simulink model "svm"  (R2021b)
settings: Solver=VariableStepAuto  StartTime=0.0  StopTime=10.0  RelTol=1e-3
libraries: spsIGBTDiodeLib x6, slpidlib x2, spsAsynchronousMachineSIUnitsLib x1, spsDCVoltageSourceLib x1, mcbcontrolslib x1, simulink_extras x1, spsSeriesRLCBranchLib x1, spsTriangleGeneratorLib x1, spsVoltageMeasurementLib x1, spspowerguiLib x1
settings Model: Creator=borutzki  LastModifiedBy=borutzki

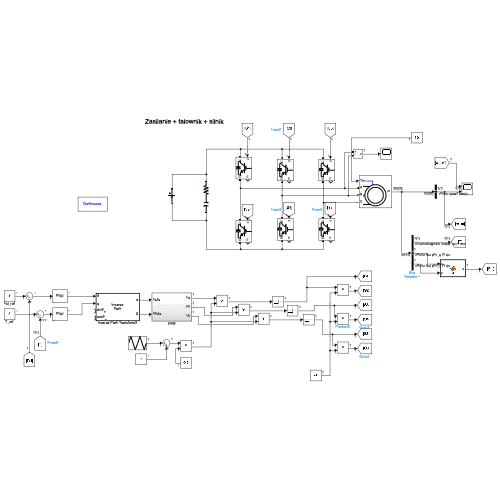
[thumbnail: Simulink's stored preview of the top-level diagram]
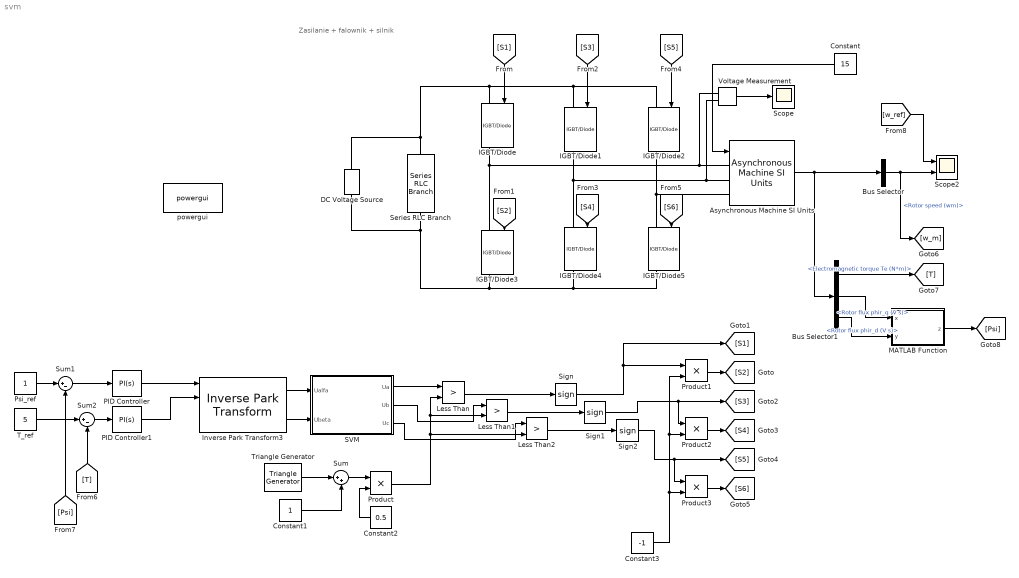
== system svm ==
  note: Zasilanie + falownik + silnik
  Asynchronous Machine SI Units : spsAsynchronousMachineSIUnitsLib/Asynchronous Machine SI Units  RotorType=Squirrel-cage  PresetModel=No  MechanicalLoad=Torque Tm  ShowDetailedParameters=on  ReferenceFrame=Rotor  Units=SI  MeasurementBus=off  NominalParameters=[1.845e+04 400 50]  VoltageRatio=1  Stator=[0.5968 0.0003495]  Rotor=[0.6258 0.005473]  Cage1=[0.4155 0.002066]  Cage2=[0.4168 0.0003495]  Lm=0.0354  Mechanical=[0.05 0.005879 2]  PolePairs=2  InitialConditions=[0 0 0 0 0 0 0 0]  SimulateSaturation=off  Saturation=[14.03593122, 27.81365428, 53.79336849, 72.68890987, 97.98006896, 148.6815601, 215.7428561, 302.9841135, 428.7778367 ; 230, 322, 414, 460, 506, 552, 598, 644, 690]  LoadFlowParameters=1492000  TsPowergui=0  TsBlock=-1  IterativeModel=Trapezoidal non iterative  IterativeDiscreteModel=Trapezoidal non iterative  Pmec=1.492e+006
  Bus Selector : BusSelector  OutputSignals=Mechanical.Rotor speed (wm)
  Bus Selector1 : BusSelector  OutputSignals=Mechanical.Electromagnetic torque Te (N*m),Rotor measurements.Rotor flux phir_q (V s),Rotor measurements.Rotor flux phir_d (V s)
  Constant : Constant  Value=15
  Constant1 : Constant
  Constant2 : Constant  Value=0.5
  Constant3 : Constant  Value=-1
  DC Voltage Source : spsDCVoltageSourceLib/DC Voltage Source  Amplitude=400  Measurements=None
  IGBT/Diode{,1..5} (6 alike) : spsIGBTDiodeLib/IGBT//Diode  Ron=1e-3  Rs=1e5  Cs=inf  Measurements=on
  Inverse Park Transform3 : mcbcontrolslib/Inverse Park Transform  AxisAlignment=D-axis
  Less Than : RelationalOperator  Operator=>  OutDataTypeStr=boolean  RndMeth=Simplest
  Less Than1 : RelationalOperator  Operator=>  OutDataTypeStr=boolean  RndMeth=Simplest
  Less Than2 : RelationalOperator  Operator=>  OutDataTypeStr=boolean  RndMeth=Simplest
  MATLAB Function : MATLAB Function  TreatAsAtomicUnit=on
  PID Controller : slpidlib/PID Controller  Controller=PI  Form=Parallel  TimeDomain=Continuous-time  UseExternalTs=off  SampleTime=-1  IntegratorMethod=Forward Euler  FilterMethod=Forward Euler  ControllerParametersSource=internal  P=1  I=1  D=0  UseFilter=on  N=100  TunerSelectOption=Transfer Function Based (PID Tuner App)  InitialConditionSource=internal  InitialConditionForIntegrator=0  InitialConditionForFilter=0  DifferentiatorICPrevScaledInput=0  ExternalReset=none  TrackingMode=off  Kt=1  LimitOutput=off  SatLimitsSource=internal  UpperSaturationLimit=inf  LowerSaturationLimit=-inf  LinearizeAsGain=on  AntiWindupMode=none  Kb=1  POutMin=[]  POutMax=[]  IOutMin=[]  IOutMax=[]  DOutMin=[]  DOutMax=[]  NOutMin=[]  NOutMax=[]  SumOutMin=[]  SumOutMax=[]  SaturationOutMin=[]  SaturationOutMax=[]  PParamMin=[]  PParamMax=[]  IParamMin=[]  IParamMax=[]  DParamMin=[]  DParamMax=[]  NParamMin=[]  NParamMax=[]  KbParamMin=[]  KbParamMax=[]  KtParamMin=[]  KtParamMax=[]  KbOutMin=[]  KbOutMax=[]  KtOutMin=[]  KtOutMax=[]  IntegratorOutMin=[]  IntegratorOutMax=[]  FilterOutMin=[]  FilterOutMax=[]  SumI1OutMin=[]  SumI1OutMax=[]  SumI2OutMin=[]  SumI2OutMax=[]  SumI3OutMin=[]  SumI3OutMax=[]  SumI4OutMin=[]  SumI4OutMax=[]  SumDOutMin=[]  SumDOutMax=[]  DifferentiatorOutMin=[]  DifferentiatorOutMax=[]  FilterDiffOutCoefMin=[]  FilterDiffOutCoefMax=[]  ReciprocalOutMin=[]  ReciprocalOutMax=[]  SumDenOutMin=[]  SumDenOutMax=[]  SumNumOutMin=[]  SumNumOutMax=[]  DivideOutMin=[]  DivideOutMax=[]  UdiffTsProdOutMin=[]  UdiffTsProdOutMax=[]  NTsProdOutMin=[]  NTsProdOutMax=[]  UintegralTsProdOutMin=[]  UintegralTsProdOutMax=[]  UngainTsProdOutMin=[]  UngainTsProdOutMax=[]  IntegratorContinuousStateAttributes=''  IntegratorStateMustResolveToSignalObject=off  IntegratorRTWStateStorageClass=Auto  FilterContinuousStateAttributes=''  FilterStateMustResolveToSignalObject=off  FilterRTWStateStorageClass=Auto  ParallelPVariant=InternalParameters  IdealPVariant=Disabled  IVariant=InternalParameters  DVariant=Disabled  IntegratorVariant=Continuous  SatVariant=Disabled  AWVariant=Passthrough  PCopyVariant=Disabled  TRVariant=Disabled  FdbkBlocksVariant=Forward  IdealPFdbkVariant=Disabled  SatFdbkVariant=Disabled  DerivativeFilterVariant=Disabled  NVariant=Disabled  NCopyVariant=Disabled_SignalSpec  FilterICVariant=Disabled  IntegratorICVariant=InternalICs  ExternalResetVariant=Disabled  TRSumVariant=Passthrough  SumFdbkVariant=Disabled  SumVariant=Sum_PI  TsampFilterVariant=InternalTs  TsampNgainVariant=Passthrough  TsampIntegralVariant=Passthrough  ExternalSaturationOutDataTypeStr=Inherit: Same as second input
  PID Controller1 : slpidlib/PID Controller  Controller=PI  Form=Parallel  TimeDomain=Continuous-time  UseExternalTs=off  SampleTime=-1  IntegratorMethod=Forward Euler  FilterMethod=Forward Euler  ControllerParametersSource=internal  P=1  I=1  D=0  UseFilter=on  N=100  TunerSelectOption=Transfer Function Based (PID Tuner App)  InitialConditionSource=internal  InitialConditionForIntegrator=0  InitialConditionForFilter=0  DifferentiatorICPrevScaledInput=0  ExternalReset=none  TrackingMode=off  Kt=1  LimitOutput=off  SatLimitsSource=internal  UpperSaturationLimit=inf  LowerSaturationLimit=-inf  LinearizeAsGain=on  AntiWindupMode=none  Kb=1  POutMin=[]  POutMax=[]  IOutMin=[]  IOutMax=[]  DOutMin=[]  DOutMax=[]  NOutMin=[]  NOutMax=[]  SumOutMin=[]  SumOutMax=[]  SaturationOutMin=[]  SaturationOutMax=[]  PParamMin=[]  PParamMax=[]  IParamMin=[]  IParamMax=[]  DParamMin=[]  DParamMax=[]  NParamMin=[]  NParamMax=[]  KbParamMin=[]  KbParamMax=[]  KtParamMin=[]  KtParamMax=[]  KbOutMin=[]  KbOutMax=[]  KtOutMin=[]  KtOutMax=[]  IntegratorOutMin=[]  IntegratorOutMax=[]  FilterOutMin=[]  FilterOutMax=[]  SumI1OutMin=[]  SumI1OutMax=[]  SumI2OutMin=[]  SumI2OutMax=[]  SumI3OutMin=[]  SumI3OutMax=[]  SumI4OutMin=[]  SumI4OutMax=[]  SumDOutMin=[]  SumDOutMax=[]  DifferentiatorOutMin=[]  DifferentiatorOutMax=[]  FilterDiffOutCoefMin=[]  FilterDiffOutCoefMax=[]  ReciprocalOutMin=[]  ReciprocalOutMax=[]  SumDenOutMin=[]  SumDenOutMax=[]  SumNumOutMin=[]  SumNumOutMax=[]  DivideOutMin=[]  DivideOutMax=[]  UdiffTsProdOutMin=[]  UdiffTsProdOutMax=[]  NTsProdOutMin=[]  NTsProdOutMax=[]  UintegralTsProdOutMin=[]  UintegralTsProdOutMax=[]  UngainTsProdOutMin=[]  UngainTsProdOutMax=[]  IntegratorContinuousStateAttributes=''  IntegratorStateMustResolveToSignalObject=off  IntegratorRTWStateStorageClass=Auto  FilterContinuousStateAttributes=''  FilterStateMustResolveToSignalObject=off  FilterRTWStateStorageClass=Auto  ParallelPVariant=InternalParameters  IdealPVariant=Disabled  IVariant=InternalParameters  DVariant=Disabled  IntegratorVariant=Continuous  SatVariant=Disabled  AWVariant=Passthrough  PCopyVariant=Disabled  TRVariant=Disabled  FdbkBlocksVariant=Forward  IdealPFdbkVariant=Disabled  SatFdbkVariant=Disabled  DerivativeFilterVariant=Disabled  NVariant=Disabled  NCopyVariant=Disabled_SignalSpec  FilterICVariant=Disabled  IntegratorICVariant=InternalICs  ExternalResetVariant=Disabled  TRSumVariant=Passthrough  SumFdbkVariant=Disabled  SumVariant=Sum_PI  TsampFilterVariant=InternalTs  TsampNgainVariant=Passthrough  TsampIntegralVariant=Passthrough  ExternalSaturationOutDataTypeStr=Inherit: Same as second input
  Product{,1..3} (4 alike) : Product
  Psi_ref : Constant
  SVM : Subsystem
  Scope : Scope
  Scope2 : Scope  NumInputPorts=2
  Series RLC Branch : spsSeriesRLCBranchLib/Series RLC Branch  LConnTagsString=__new0  RConnTagsString=__new0  BranchType=RC  Resistance=0.001  Inductance=1e-3  SetiL0=off  InitialCurrent=0  Capacitance=600e-5  Setx0=off  InitialVoltage=0  Measurements=None
  Sign : Signum
  Sign1 : Signum
  Sign2 : Signum
  Sum : Sum  Inputs=|++
  Sum1 : Sum  Inputs=|+-
  Sum2 : Sum  Inputs=|+-
  T_ref : Constant  Value=5
  Triangle Generator : spsTriangleGeneratorLib/Triangle Generator  Freq=5e3  Phase=90  Ts=0
  Voltage Measurement : spsVoltageMeasurementLib/Voltage Measurement  PhasorSimulation=off  OutputType=Complex  PSBequivalent=0
  powergui : spspowerguiLib/powergui  Priority=1  SimulationMode=Continuous  SampleTime=50e-6  frequency=60  Iterations=50  frequencyindice=50  Pbase=100e6  ErrMax=1e-4  UnitsV=kV  UnitsW=MW  buscounter=0  FunctionMessages=off  echomessages=off  EnableUseOfTLC=off  CurrentSourceSwitches=off  DisableSnubberDevices=off  DisableRonSwitches=off  DisableVfSwitches=off  DisplayEquations=off  AutomaticDiscreteSolvers=off  SolverType=Tustin/Backward Euler (TBE)  Interpol=off  ExternalGateDelay=off  methode=off  Ts=100  x0status=blocks  SPID=on  SwTol=0  HookPort=off  NonlinearTolerance=1e-4  nMaxIteration=100  ContinueOnMaxIteration=off  RestoreLinks=warning  ResistiveCurrentMeasurement=off  Frange=[0:2:500]  Ylog=off  Xlog=on  ShowGrid=off  save=off  variable=ZData  structure=0  ZoomFFT=off  StartTime=0.0  cycles=1  DisplayStyle=1  fundamental=60  FreqAxis=off  MaxFrequency=1000  frequencyindicesteady=1  RmsSteady=1  display=off
  wires:
  [S4] -> IGBT/Diode4/1
  Voltage Measurement/1 -> Scope/1
  [S5] -> IGBT/Diode2/1
  [S6] -> IGBT/Diode5/1
  Asynchronous Machine SI Units/1 -> Bus Selector1/1, Bus Selector/1
  [S3] -> IGBT/Diode1/1
  [S2] -> IGBT/Diode3/1
  [S1] -> IGBT/Diode/1
  Bus Selector/1 -> [w_m], Scope2/2  "<Rotor speed (wm)>"
  [w_ref] -> Scope2/1
  Constant/1 -> Asynchronous Machine SI Units/1
  Constant1/1 -> Sum/2
  Triangle Generator/1 -> Sum/1
  Sum/1 -> Product/1
  Constant2/1 -> Product/2
  SVM/1(Ua) -> Less Than/1
  SVM/2(Ub) -> Less Than1/1
  SVM/3(Uc) -> Less Than2/1
  Product/1 -> Less Than2/2, Less Than/2, Less Than1/2
  Less Than/1 -> Sign/1
  Less Than1/1 -> Sign1/1
  Less Than2/1 -> Sign2/1
  Product1/1 -> [S2]
  Product2/1 -> [S4]
  Product3/1 -> [S6]
  Constant3/1 -> Product1/2, Product2/2, Product3/2
  Sign/1 -> [S1], Product1/1
  Sign1/1 -> Product2/1, [S3]
  Sign2/1 -> Product3/1, [S5]
  Inverse Park Transform3/1 -> SVM/1(Ualfa)
  Inverse Park Transform3/2 -> SVM/2(Ubeta)
  Sum2/1 -> PID Controller1/1
  Sum1/1 -> PID Controller/1
  Psi_ref/1 -> Sum1/1
  T_ref/1 -> Sum2/1
  Bus Selector1/1 -> [T]  "<Electromagnetic torque Te (N*m)>"
  [T] -> Sum2/2
  Bus Selector1/2 -> MATLAB Function/1(x)  "<Rotor flux phir_q (V s)>"
  Bus Selector1/3 -> MATLAB Function/2(y)  "<Rotor flux phir_d (V s)>"
  MATLAB Function/1(z) -> [Psi]
  [Psi] -> Sum1/2
  PID Controller1/1 -> Inverse Park Transform3/2
  PID Controller/1 -> Inverse Park Transform3/1
  connections:
  IGBT/Diode2/RConn1 -- Asynchronous Machine SI Units/LConn3 -- IGBT/Diode5/LConn1
  IGBT/Diode/RConn1 -- Asynchronous Machine SI Units/LConn1 -- Voltage Measurement/LConn1 -- IGBT/Diode3/LConn1
  IGBT/Diode1/LConn1 -- IGBT/Diode2/LConn1 -- IGBT/Diode/LConn1 -- Series RLC Branch/LConn1 -- DC Voltage Source/RConn1
  IGBT/Diode4/RConn1 -- DC Voltage Source/LConn1 -- Series RLC Branch/RConn1 -- IGBT/Diode3/RConn1 -- IGBT/Diode5/RConn1
  IGBT/Diode1/RConn1 -- Asynchronous Machine SI Units/LConn2 -- Voltage Measurement/LConn2 -- IGBT/Diode4/LConn1

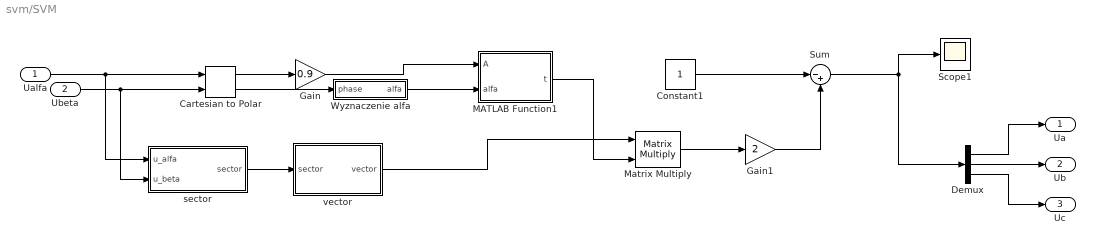
== system svm/SVM ==
  Ualfa : Inport
  Ubeta : Inport  Port=2
  Cartesian to Polar : simulink_extras/Transformations/Cartesian to Polar
  Constant1 : Constant
  Demux : Demux  Outputs=3
  Gain : Gain  Gain=0.9
  Gain1 : Gain  Gain=2
  MATLAB Function1 : MATLAB Function  TreatAsAtomicUnit=on
  Matrix Multiply : Product  Multiplication=Matrix(*)
  Scope1 : Scope
  Sum : Sum  Inputs=|-+
  Wyznaczenie alfa : MATLAB Function  TreatAsAtomicUnit=on
  sector : MATLAB Function  TreatAsAtomicUnit=on
  vector : MATLAB Function  TreatAsAtomicUnit=on
  Ua : Outport
  Ub : Outport  Port=2
  Uc : Outport  Port=3
  wires:
  Demux/1 -> Ua/1
  Gain1/1 -> Sum/2
  Constant1/1 -> Sum/1
  Cartesian to Polar/1 -> Gain/1
  Matrix Multiply/1 -> Gain1/1
  Ualfa/1 -> sector/1(u_alfa), Cartesian to Polar/1
  MATLAB Function1/1(t) -> Matrix Multiply/2
  vector/1(vector) -> Matrix Multiply/1
  Ubeta/1 -> Cartesian to Polar/2, sector/2(u_beta)
  Gain/1 -> MATLAB Function1/1(A)
  Demux/3 -> Uc/1
  Cartesian to Polar/2 -> Wyznaczenie alfa/1(phase)
  Demux/2 -> Ub/1
  Sum/1 -> Demux/1, Scope1/1
  sector/1(sector) -> vector/1(sector)
  Wyznaczenie alfa/1(alfa) -> MATLAB Function1/2(alfa)

== matlab function svm/MATLAB Function ==
  data: x input; z output; y input
function z = fcn(x,y)

z = sqrt(x^2+y^2);

== matlab function svm/SVM/vector ==
  data: sector input; vector output
function vector = fcn(sector)
switch sector
    case 1
        vector = [1 1 0.5; 0 1 0.5; 0 0 0.5];
    case 2
        vector = [1 0 0.5; 1 1 0.5; 0 0 0.5];
    case 3
        vector = [0 0 0.5; 1 1 0.5; 0 1 0.5];
    case 4
        vector = [0 0 0.5; 1 0 0.5; 1 1 0.5];
    case 5
        vector = [0 1 0.5; 0 0 0.5; 1 1 0.5];
    case 6
        vector = [1 1 0.5; 0 0 0.5; 1 0 0.5];
    otherwise
        vector = [0 0 0; 0 0 0; 0 0 0];
end

== matlab function svm/SVM/Wyznaczenie alfa ==
  data: phase input; alfa output
function alfa = fcn(phase)

alfa = mod(phase,pi/3);

== matlab function svm/SVM/MATLAB Function1 ==
  data: A input; t output; alfa input
function t = fcn(A, alfa)
t1 = A*sin(pi/3 - alfa);
t2 = A*sin(alfa);
t3 = 1 - t1 - t2;
t = [t1 t2 t3];

== matlab function svm/SVM/sector ==
  data: u_alfa input; sector output; u_beta input
function sector = fcn(u_alfa,u_beta)
theta_ref = atan(u_beta/u_alfa);
sector = int(theta_ref/(pi/3))+1;
